simulink model "lump_model_v3"  (R2024b)
settings: Solver=VariableStepAuto  StartTime=0.0  StopTime=66  RelTol=1e-3
model workspace (MAT data in the model file):
  A_busbar = 0.0015
  A_pack = 0.711626248
  C_nominal = 3
  I_max = 157.708978328
  P = 5
  S = 138
  SoC_initial = 1
  T_amb = 301.15
  busbar_CC_area = 0.000108
  busbar_Cp = 237
  busbar_length = 0.032
  busbar_mass = 0.01
  busbar_resistivity = 1.68e-08
  busbar_thermalcontact_resistance = 1
  cell_Cp = 1000
  cell_mass = 0.046
  h_busbar = 5
  h_pack = 7.83952040581
(part 1 of 3)
settings Model: Creator=kara.28  LastModifiedBy=kara.28

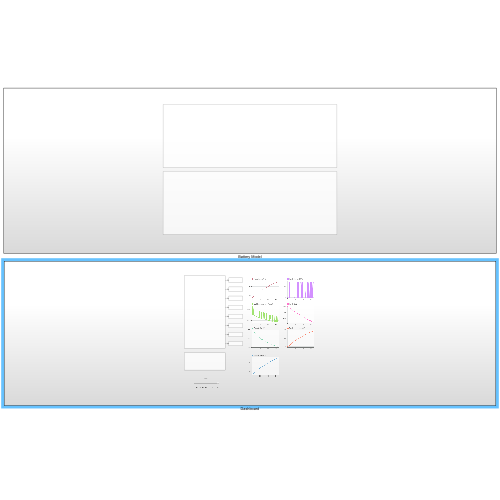
[thumbnail: Simulink's stored preview of the top-level diagram]
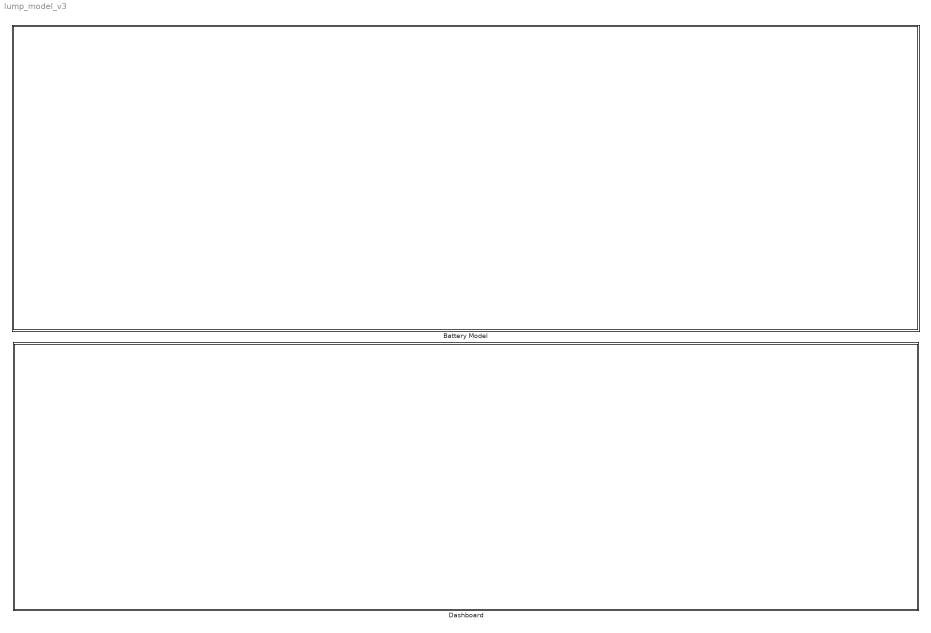
== system lump_model_v3 ==
  Battery Model : Subsystem
  Dashboard : Subsystem

== system lump_model_v3/Battery Model ==
  Battery Cells : Subsystem
  Busbars : Subsystem

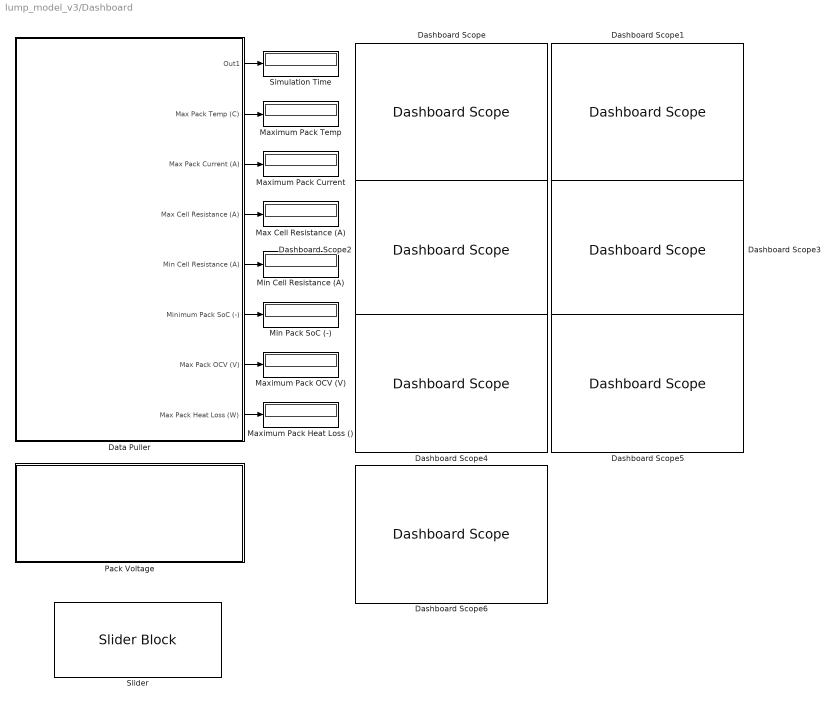
== system lump_model_v3/Dashboard ==
  Dashboard Scope : DashboardScope  Ymin=0  Ymax=100
  Dashboard Scope{1..6} (6 alike) : DashboardScope
  Data Puller : Subsystem
  Max Cell Resistance (A) : Display
  Maximum Pack Current : Display
  Maximum Pack Heat Loss () : Display
  Maximum Pack OCV (V) : Display
  Maximum Pack Temp : Display
  Min Cell Resistance (A) : Display
  Min Pack SoC (-) : Display
  Pack Voltage : Subsystem
  Simulation Time : Display
  Slider : SliderBlock  ScaleMax=160
  wires:
  Data Puller/1(Out1) -> Simulation Time/1
  Data Puller/2(Max Pack Temp (C)) -> Maximum Pack Temp/1
  Data Puller/3(Max Pack Current (A)) -> Maximum Pack Current/1
  Data Puller/4(Max Cell Resistance (A)) -> Max Cell Resistance (A)/1
  Data Puller/5(Min Cell Resistance (A)) -> Min Cell Resistance (A)/1
  Data Puller/6(Minimum Pack SoC (-)) -> Min Pack SoC (-)/1
  Data Puller/7(Max Pack OCV (V)) -> Maximum Pack OCV (V)/1
  Data Puller/8(Max Pack Heat Loss (W)) -> Maximum Pack Heat Loss ()/1

== system lump_model_v3/Battery Model/Battery Cells ==
  Battery Heat : Subsystem
      settings: PortSchema="{\"entries\":[{\"content\":{\"sides\":[{\"content\":{\"connectorIds\":[\"In1\",\"Out1\",\"In2\",\"In3\"]},\"type\":\"ConnectorPlacement.EquallySpacedRectSide\",\"uuid\":\"0f7c0562-63f7-413a-9c65-7d5d0f23ac53\"},{\"content\":{\"side\":\"RIGHT\"},\"type\":\"ConnectorPlacement.EquallySpacedRectSide\",\"uuid\":\"6856fc4a-e601-47fb-aafe-3183d6398fa2\"},{\"content\":{\"side\":\"TOP\"},\"type\":\"ConnectorPlacement.EquallySpacedRectSide\",\"uuid\":\"93500152-ab0c-4e86-a765-8796b82b9cd6\"}]},\"type\":\"ConnectorPlacement.EquallySpacedConnector\",\"uuid\":\"8bef09a8-0835-4033-ba4e-3f5f6277d0ac\"}],\"packageUris\":[\"http://schema.mathworks.com/mf0/Connector/R2020b\"],\"version\":\"1.0\"}"
  Battery Heat Generation : Subsystem
  Busbar - Segment Heat Flow : Subsystem
      settings: PortSchema="{\"entries\":[{\"content\":{\"sides\":[{\"content\":{},\"type\":\"ConnectorPlacement.EquallySpacedRectSide\",\"uuid\":\"839c7b7c-3d90-4543-803d-828e2cd8ee3e\"},{\"content\":{\"connectorIds\":[\"In1\",\"Out1\"],\"side\":\"RIGHT\"},\"type\":\"ConnectorPlacement.EquallySpacedRectSide\",\"uuid\":\"e3492608-3f40-473c-8392-0c925b682872\"},{\"content\":{\"side\":\"TOP\"},\"type\":\"ConnectorPlacement.EquallySpacedRectSide\",\"uuid\":\"8e15337c-e61d-491c-b508-620217c9bb60\"}]},\"type\":\"ConnectorPlacement.EquallySpacedConnector\",\"uuid\":\"03d3ec16-7a24-4203-9805-446eb586226e\"}],\"packageUris\":[\"http://schema.mathworks.com/mf0/Connector/R2020b\"],\"version\":\"1.0\"}"
  Heat Loss : Subsystem
      settings: PortSchema="{\"entries\":[{\"content\":{\"sides\":[{\"content\":{},\"type\":\"ConnectorPlacement.EquallySpacedRectSide\",\"uuid\":\"cd11f8f0-ebc0-4dda-8c98-00f5919de41a\"},{\"content\":{\"connectorIds\":[\"In1\",\"Out1\"],\"side\":\"RIGHT\"},\"type\":\"ConnectorPlacement.EquallySpacedRectSide\",\"uuid\":\"2a68a9a1-bd97-4a17-8a8b-1aa98e9bd9a8\"},{\"content\":{\"side\":\"TOP\"},\"type\":\"ConnectorPlacement.EquallySpacedRectSide\",\"uuid\":\"debcc510-941b-4448-a371-f67c84c59f32\"}]},\"type\":\"ConnectorPlacement.EquallySpacedConnector\",\"uuid\":\"91559e46-754b-48b4-ac3e-ab135f9add0a\"}],\"packageUris\":[\"http://schema.mathworks.com/mf0/Connector/R2020b\"],\"version\":\"1.0\"}"
  wires:
  Battery Heat/1(Pack Temp (K)) -> Busbar - Segment Heat Flow/1(Segment Temp (K)), Heat Loss/1(Pack Temp (K))
  Battery Heat Generation/1(Battery Heat Generation Rate) -> Battery Heat/1(Battery Heat Generation)
  Heat Loss/1(Pack Heat Loss Rate) -> Battery Heat/2(Battery Heat Loss)
  Busbar - Segment Heat Flow/1(Busbar - Segment Heat Flow (W)) -> Battery Heat/3(Busbar - Segment Heat Flow (W))

== system lump_model_v3/Battery Model/Busbars ==
  Ambient Heat Loss : Subsystem
      settings: PortSchema="{\"entries\":[{\"content\":{\"sides\":[{\"content\":{},\"type\":\"ConnectorPlacement.EquallySpacedRectSide\",\"uuid\":\"cd11f8f0-ebc0-4dda-8c98-00f5919de41a\"},{\"content\":{\"connectorIds\":[\"In1\",\"Out1\"],\"side\":\"RIGHT\"},\"type\":\"ConnectorPlacement.EquallySpacedRectSide\",\"uuid\":\"2a68a9a1-bd97-4a17-8a8b-1aa98e9bd9a8\"},{\"content\":{\"side\":\"TOP\"},\"type\":\"ConnectorPlacement.EquallySpacedRectSide\",\"uuid\":\"debcc510-941b-4448-a371-f67c84c59f32\"}]},\"type\":\"ConnectorPlacement.EquallySpacedConnector\",\"uuid\":\"91559e46-754b-48b4-ac3e-ab135f9add0a\"}],\"packageUris\":[\"http://schema.mathworks.com/mf0/Connector/R2020b\"],\"version\":\"1.0\"}"
  Busbar - Segment Heat Flow : Subsystem
      settings: PortSchema="{\"entries\":[{\"content\":{\"sides\":[{\"content\":{},\"type\":\"ConnectorPlacement.EquallySpacedRectSide\",\"uuid\":\"839c7b7c-3d90-4543-803d-828e2cd8ee3e\"},{\"content\":{\"connectorIds\":[\"In1\",\"Out1\"],\"side\":\"RIGHT\"},\"type\":\"ConnectorPlacement.EquallySpacedRectSide\",\"uuid\":\"e3492608-3f40-473c-8392-0c925b682872\"},{\"content\":{\"side\":\"TOP\"},\"type\":\"ConnectorPlacement.EquallySpacedRectSide\",\"uuid\":\"8e15337c-e61d-491c-b508-620217c9bb60\"}]},\"type\":\"ConnectorPlacement.EquallySpacedConnector\",\"uuid\":\"03d3ec16-7a24-4203-9805-446eb586226e\"}],\"packageUris\":[\"http://schema.mathworks.com/mf0/Connector/R2020b\"],\"version\":\"1.0\"}"
  Busbar Heat : Subsystem
      settings: PortSchema="{\"entries\":[{\"content\":{\"sides\":[{\"content\":{\"connectorIds\":[\"In1\",\"Out1\",\"In2\",\"In3\"]},\"type\":\"ConnectorPlacement.EquallySpacedRectSide\",\"uuid\":\"0f7c0562-63f7-413a-9c65-7d5d0f23ac53\"},{\"content\":{\"side\":\"RIGHT\"},\"type\":\"ConnectorPlacement.EquallySpacedRectSide\",\"uuid\":\"6856fc4a-e601-47fb-aafe-3183d6398fa2\"},{\"content\":{\"side\":\"TOP\"},\"type\":\"ConnectorPlacement.EquallySpacedRectSide\",\"uuid\":\"93500152-ab0c-4e86-a765-8796b82b9cd6\"}]},\"type\":\"ConnectorPlacement.EquallySpacedConnector\",\"uuid\":\"8bef09a8-0835-4033-ba4e-3f5f6277d0ac\"}],\"packageUris\":[\"http://schema.mathworks.com/mf0/Connector/R2020b\"],\"version\":\"1.0\"}"
  Resistance Heat Generation : Subsystem
  wires:
  Busbar Heat/1(Busbar Temp (K)) -> Busbar - Segment Heat Flow/1(Busbar Temp (K)), Ambient Heat Loss/1(Busbar Temp (K))
  Resistance Heat Generation/1(Busbar Heat Generation Rate) -> Busbar Heat/1(Busbar Heat Generation)
  Ambient Heat Loss/1(Busbar Heat Loss Rate) -> Busbar Heat/2(Busbar Heat Loss)
  Busbar - Segment Heat Flow/1(Busbar - Segment Heat Flow (W)) -> Busbar Heat/3(Busbar - Segment Heat Flow (W))

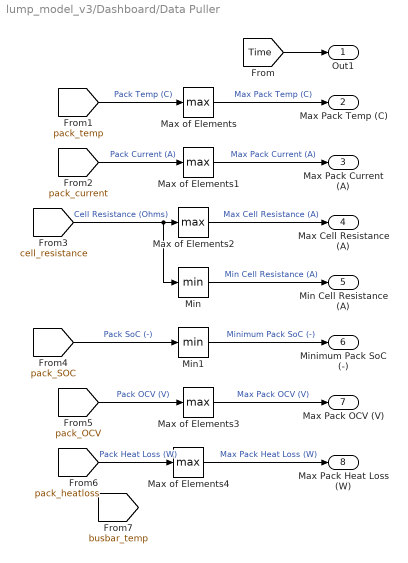
== system lump_model_v3/Dashboard/Data Puller ==
  Max of Elements{,1..4} (5 alike) : MinMax  Function=max
  Min : MinMax
  Min1 : MinMax
  Out1 : Outport
  Max Pack Temp (C) : Outport  Port=2
  Max Pack Current (A) : Outport  Port=3
  Max Cell Resistance (A) : Outport  Port=4
  Min Cell Resistance (A) : Outport  Port=5
  Minimum Pack SoC (-) : Outport  Port=6
  Max Pack OCV (V) : Outport  Port=7
  Max Pack Heat Loss (W) : Outport  Port=8
  wires:
  Min1/1 -> Minimum Pack SoC (-)/1  "Minimum Pack SoC (-)"
  [pack_current] -> Max of Elements1/1  "Pack Current (A)"
  [cell_resistance] -> Min/1, Max of Elements2/1  "Cell Resistance (Ohms)"
  [pack_heatloss] -> Max of Elements4/1  "Pack Heat Loss (W)"
  [pack_temp] -> Max of Elements/1  "Pack Temp (C)"
  [pack_OCV] -> Max of Elements3/1  "Pack OCV (V)"
  [pack_SOC] -> Min1/1  "Pack SoC (-)"
  Max of Elements1/1 -> Max Pack Current (A)/1  "Max Pack Current (A)"
  Max of Elements2/1 -> Max Cell Resistance (A)/1  "Max Cell Resistance (A)"
  Max of Elements/1 -> Max Pack Temp (C)/1  "Max Pack Temp (C)"
  Max of Elements4/1 -> Max Pack Heat Loss (W)/1  "Max Pack Heat Loss (W)"
  Max of Elements3/1 -> Max Pack OCV (V)/1  "Max Pack OCV (V)"
  [Time] -> Out1/1
  Min/1 -> Min Cell Resistance (A)/1  "Min Cell Resistance (A)"

== system lump_model_v3/Dashboard/Pack Voltage ==
  Gain : Gain  Gain=S
  Lookup with Linear Lagrange Interpolation : Lookup_n-D  NumberOfTableDimensions=1  BreakpointsForDimension1=[0.100961;0.201247;0.30155;0.401865;0.502237;0.602602;0.7029339999999999;0.8032629999999999;0.903617;1]  Table=[3.227877;3.437376;3.537935;3.663634;3.755814;3.835423;3.940172;4.047017;4.097296;4.187904]  InterpMethod=Cubic spline  InternalRulePriority=Speed  RndMeth=Simplest
  tag scope: pack_OCV=global
  wires:
  [pack_SOC] -> Lookup with Linear Lagrange Interpolation/1
  Lookup with Linear Lagrange Interpolation/1 -> Gain/1
  Gain/1 -> [pack_OCV]  "Pack OCV (V)"

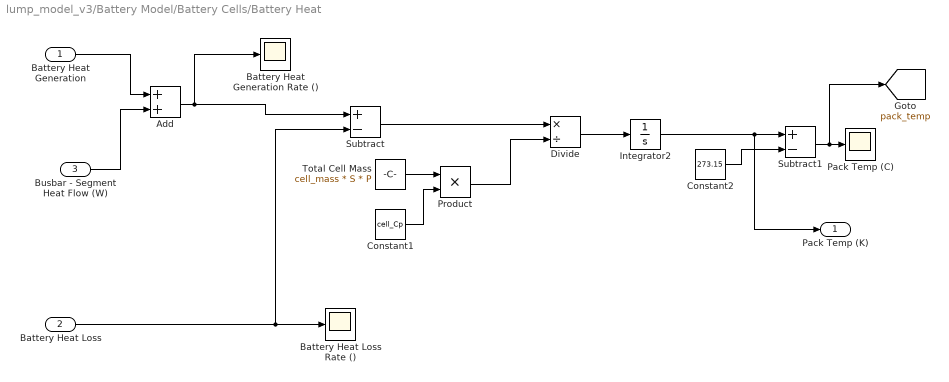
== system lump_model_v3/Battery Model/Battery Cells/Battery Heat ==
  Battery Heat Generation : Inport
  Battery Heat Loss : Inport  Port=2
  Busbar - Segment Heat Flow (W) : Inport  Port=3
  Add : Sum
  Battery Heat Generation Rate () : Scope
  Battery Heat Loss Rate () : Scope
  Constant1 : Constant  Value=cell_Cp
  Constant2 : Constant  Value=273.15
  Divide : Product  Inputs=*/
  Integrator2 : Integrator  InitialCondition=T_amb
  Pack Temp (C) : Scope
  Product : Product
  Subtract : Sum  Inputs=+-
  Subtract1 : Sum  Inputs=+-
  Total Cell Mass : Constant  Value=cell_mass * S * P
  Pack Temp (K) : Outport
  tag scope: pack_temp=global
  wires:
  Constant1/1 -> Product/2
  Constant2/1 -> Subtract1/2
  Divide/1 -> Integrator2/1
  Subtract/1 -> Divide/1
  Integrator2/1 -> Pack Temp (K)/1, Subtract1/1
  Subtract1/1 -> [pack_temp], Pack Temp (C)/1
  Total Cell Mass/1 -> Product/1
  Product/1 -> Divide/2
  Battery Heat Loss/1 -> Battery Heat Loss Rate ()/1, Subtract/2
  Battery Heat Generation/1 -> Add/1
  Busbar - Segment Heat Flow (W)/1 -> Add/2
  Add/1 -> Subtract/1, Battery Heat Generation Rate ()/1

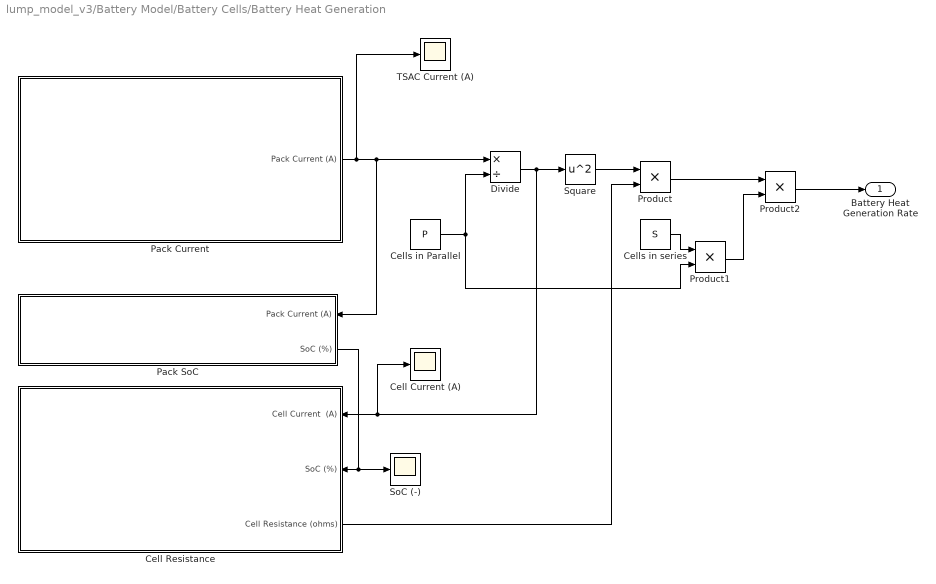
== system lump_model_v3/Battery Model/Battery Cells/Battery Heat Generation ==
  Cell Current (A) : Scope
  Cell Resistance : Subsystem
      settings: PortSchema="{\"entries\":[{\"content\":{\"sides\":[{\"content\":{},\"type\":\"ConnectorPlacement.EquallySpacedRectSide\",\"uuid\":\"1c6ff2a8-2c86-4b92-aa7d-5717a02d6f28\"},{\"content\":{\"connectorIds\":[\"In1\",\"In2\",\"Out1\"],\"side\":\"RIGHT\"},\"type\":\"ConnectorPlacement.EquallySpacedRectSide\",\"uuid\":\"52a4cb2c-e1db-459d-bd0a-206cc3bba6d1\"},{\"content\":{\"side\":\"TOP\"},\"type\":\"ConnectorPlacement.EquallySpacedRectSide\",\"uuid\":\"751bbbd6-abc7-4265-8d68-4aa70d69379f\"}]},\"type\":\"ConnectorPlacement.EquallySpacedConnector\",\"uuid\":\"b8f9630f-0167-4478-8d98-637e13782dcd\"}],\"packageUris\":[\"http://schema.mathworks.com/mf0/Connector/R2020b\"],\"version\":\"1.0\"}"
  Cells in Parallel : Constant  Value=P
  Cells in series : Constant  Value=S
  Divide : Product  Inputs=*/
  Pack Current : Subsystem
  Pack SoC : Subsystem
      settings: PortSchema="{\"entries\":[{\"content\":{\"sides\":[{\"content\":{},\"type\":\"ConnectorPlacement.EquallySpacedRectSide\",\"uuid\":\"1c6ff2a8-2c86-4b92-aa7d-5717a02d6f28\"},{\"content\":{\"connectorIds\":[\"In1\",\"Out1\"],\"side\":\"RIGHT\"},\"type\":\"ConnectorPlacement.EquallySpacedRectSide\",\"uuid\":\"52a4cb2c-e1db-459d-bd0a-206cc3bba6d1\"},{\"content\":{\"side\":\"TOP\"},\"type\":\"ConnectorPlacement.EquallySpacedRectSide\",\"uuid\":\"751bbbd6-abc7-4265-8d68-4aa70d69379f\"}]},\"type\":\"ConnectorPlacement.EquallySpacedConnector\",\"uuid\":\"b8f9630f-0167-4478-8d98-637e13782dcd\"}],\"packageUris\":[\"http://schema.mathworks.com/mf0/Connector/R2020b\"],\"version\":\"1.0\"}"
  Product : Product
  Product1 : Product
  Product2 : Product
  SoC (-) : Scope
  Square : Math  Operator=square
  TSAC Current (A) : Scope
  Battery Heat Generation Rate : Outport
  wires:
  Cells in series/1 -> Product1/1
  Divide/1 -> Cell Current (A)/1, Cell Resistance/1(Cell Current  (A)), Square/1
  Cell Resistance/1(Cell Resistance (ohms)) -> Product/2
  Square/1 -> Product/1
  Cells in Parallel/1 -> Divide/2, Product1/2
  Product1/1 -> Product2/2
  Product/1 -> Product2/1
  Product2/1 -> Battery Heat Generation Rate/1
  Pack SoC/1(SoC (%)) -> SoC (-)/1, Cell Resistance/2(SoC (%))
  Pack Current/1(Pack Current (A)) -> TSAC Current (A)/1, Divide/1, Pack SoC/1(Pack Current (A))

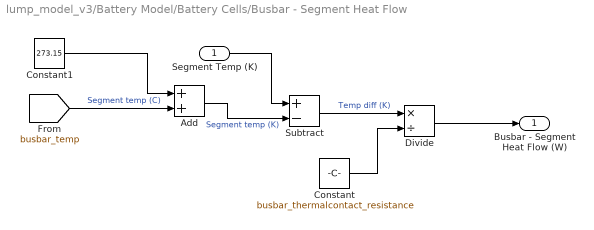
== system lump_model_v3/Battery Model/Battery Cells/Busbar - Segment Heat Flow ==
  Segment Temp (K) : Inport
  Add : Sum
  Constant : Constant  Value=busbar_thermalcontact_resistance
  Constant1 : Constant  Value=273.15
  Divide : Product  Inputs=*/
  Subtract : Sum  Inputs=+-
  Busbar - Segment Heat Flow (W) : Outport
  wires:
  Subtract/1 -> Divide/1  "Temp diff (K)"
  Constant/1 -> Divide/2
  Divide/1 -> Busbar - Segment Heat Flow (W)/1
  [busbar_temp] -> Add/2  "Segment temp (C)"
  Constant1/1 -> Add/1
  Segment Temp (K)/1 -> Subtract/1
  Add/1 -> Subtract/2  "Segment temp (K)"

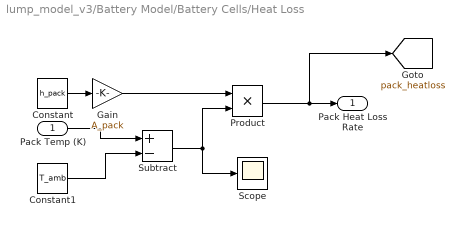
== system lump_model_v3/Battery Model/Battery Cells/Heat Loss ==
  Pack Temp (K) : Inport
  Constant : Constant  Value=h_pack
  Constant1 : Constant  Value=T_amb
  Gain : Gain  Gain=A_pack
  Product : Product
  Scope : Scope
  Subtract : Sum  Inputs=+-
  Pack Heat Loss Rate : Outport
  tag scope: pack_heatloss=global
  wires:
  Constant/1 -> Gain/1
  Subtract/1 -> Product/2, Scope/1
  Gain/1 -> Product/1
  Product/1 -> [pack_heatloss], Pack Heat Loss Rate/1
  Pack Temp (K)/1 -> Subtract/1
  Constant1/1 -> Subtract/2

== system lump_model_v3/Battery Model/Busbars/Ambient Heat Loss ==
  Busbar Temp (K) : Inport
  Constant : Constant  Value=h_busbar
  Constant1 : Constant  Value=T_amb
  Gain : Gain  Gain=A_busbar
  Product : Product
  Subtract : Sum  Inputs=+-
  Busbar Heat Loss Rate : Outport
  tag scope: busbar_heatloss=global
  wires:
  Constant/1 -> Gain/1
  Subtract/1 -> Product/2
  Gain/1 -> Product/1
  Product/1 -> [busbar_heatloss], Busbar Heat Loss Rate/1
  Busbar Temp (K)/1 -> Subtract/1
  Constant1/1 -> Subtract/2

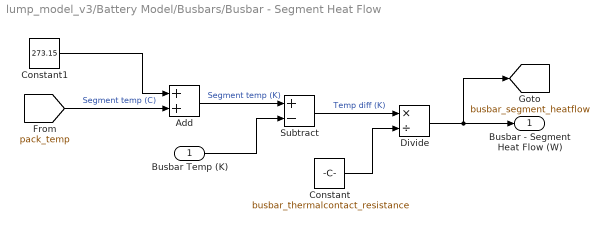
== system lump_model_v3/Battery Model/Busbars/Busbar - Segment Heat Flow ==
  Busbar Temp (K) : Inport
  Add : Sum
  Constant : Constant  Value=busbar_thermalcontact_resistance
  Constant1 : Constant  Value=273.15
  Divide : Product  Inputs=*/
  Subtract : Sum  Inputs=+-
  Busbar - Segment Heat Flow (W) : Outport
  tag scope: busbar_segment_heatflow=global
  wires:
  Busbar Temp (K)/1 -> Subtract/2
  Subtract/1 -> Divide/1  "Temp diff (K)"
  Constant/1 -> Divide/2
  Divide/1 -> [busbar_segment_heatflow], Busbar - Segment Heat Flow (W)/1
  [pack_temp] -> Add/2  "Segment temp (C)"
  Constant1/1 -> Add/1
  Add/1 -> Subtract/1  "Segment temp (K)"

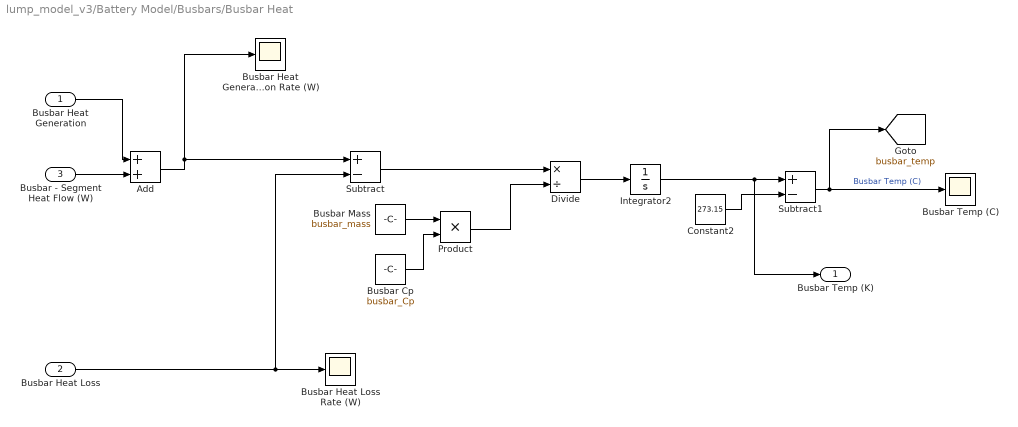
== system lump_model_v3/Battery Model/Busbars/Busbar Heat ==
  Busbar Heat Generation : Inport
  Busbar Heat Loss : Inport  Port=2
  Busbar - Segment Heat Flow (W) : Inport  Port=3
  Add : Sum
  Busbar Cp : Constant  Value=busbar_Cp
  Busbar Heat Generation Rate (W) : Scope
  Busbar Heat Loss Rate (W) : Scope
  Busbar Mass : Constant  Value=busbar_mass
  Busbar Temp (C) : Scope
  Constant2 : Constant  Value=273.15
  Divide : Product  Inputs=*/
  Integrator2 : Integrator  InitialCondition=T_amb
  Product : Product
  Subtract : Sum  Inputs=+-
  Subtract1 : Sum  Inputs=+-
  Busbar Temp (K) : Outport
  tag scope: busbar_temp=global
  wires:
  Busbar Cp/1 -> Product/2
  Constant2/1 -> Subtract1/2
  Busbar Heat Generation/1 -> Add/1
  Divide/1 -> Integrator2/1
  Subtract/1 -> Divide/1
  Integrator2/1 -> Busbar Temp (K)/1, Subtract1/1
  Subtract1/1 -> [busbar_temp], Busbar Temp (C)/1  "Busbar Temp (C)"
  Busbar Mass/1 -> Product/1
  Product/1 -> Divide/2
  Busbar Heat Loss/1 -> Busbar Heat Loss Rate (W)/1, Subtract/2
  Busbar - Segment Heat Flow (W)/1 -> Add/2
  Add/1 -> Subtract/1, Busbar Heat Generation Rate (W)/1

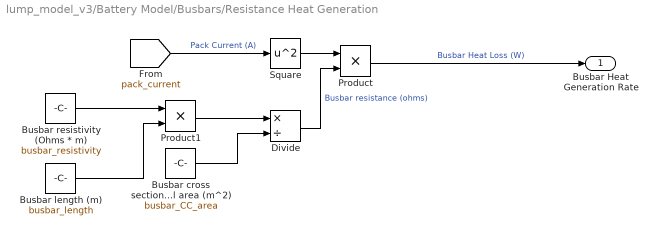
== system lump_model_v3/Battery Model/Busbars/Resistance Heat Generation ==
  Busbar cross sectional area (m^2) : Constant  Value=busbar_CC_area
  Busbar length (m) : Constant  Value=busbar_length
  Busbar resistivity (Ohms * m) : Constant  Value=busbar_resistivity
  Divide : Product  Inputs=*/
  Product : Product
  Product1 : Product
  Square : Math  Operator=square
  Busbar Heat Generation Rate : Outport
  wires:
  Product/1 -> Busbar Heat Generation Rate/1  "Busbar Heat Loss (W)"
  [pack_current] -> Square/1  "Pack Current (A)"
  Square/1 -> Product/1
  Busbar resistivity (Ohms * m)/1 -> Product1/1
  Busbar length (m)/1 -> Product1/2
  Product1/1 -> Divide/1
  Busbar cross sectional area (m^2)/1 -> Divide/2
  Divide/1 -> Product/2  "Busbar resistance (ohms)"

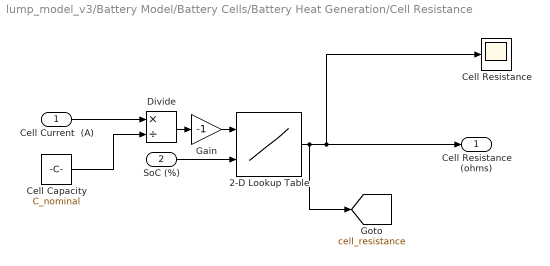
== system lump_model_v3/Battery Model/Battery Cells/Battery Heat Generation/Cell Resistance ==
  Cell Current  (A) : Inport
  SoC (%) : Inport  Port=2
  2-D Lookup Table : Lookup_n-D  BreakpointsForDimension1=[-10;-5;-1;1;2;3]  BreakpointsForDimension2=[0.1;0.2;0.3;0.4;0.5;0.6;0.7;0.8;0.9;1]  Table=[0.018906 0.01868 0.018453 0.018226 0.017999 0.017916 0.017743 0.018183 0.019549 0.022703;0.021356 0.020344 0.019332 0.019017 0.018694 0.018598 0.018319 0.018773 0.020642 0.024917;0.02305 0.020909 0.018859 0.019644 0.019687 0.018989 0.018291 0.019295 0.021608 0.026536;0.023001 0.020599 0.019683 0.019161 0.01894 0.018506 0.018636 0.019336 0.020993 0.02265;0.022654 0.020712 0.018901 0.018682 0.018442 0.018289 0.017788 0.017286 0.016785 0.016283;0.019898 0.017891 0.017366 0.01725 0.01725 0.017251 0.017251 0.017251 0.017251 0.017251]  InterpMethod=Cubic spline  ExtrapMethod=Clip  InternalRulePriority=Speed  RndMeth=Simplest
      settings: InputPortMap=u0,u1
  Cell Capacity : Constant  Value=C_nominal
  "Cell Resistance " : Scope
  Divide : Product  Inputs=*/
  Gain : Gain  Gain=-1
  Cell Resistance (ohms) : Outport
  tag scope: cell_resistance=global
  wires:
  Cell Current  (A)/1 -> Divide/1
  Cell Capacity/1 -> Divide/2
  SoC (%)/1 -> 2-D Lookup Table/2
  2-D Lookup Table/1 -> "Cell Resistance "/1, Cell Resistance (ohms)/1, [cell_resistance]
  Divide/1 -> Gain/1
  Gain/1 -> 2-D Lookup Table/1
